simulink model "One_Phase_Controlled_Thyristor_Rectifier"  (R2015a)
settings: Solver=ode45  StartTime=0.0  StopTime=1  RelTol=1e-3
libraries: powerlib x29, powerlib_meascontrol x6
settings Model: Creator=Koustubh  LastModifiedBy=Koustubh

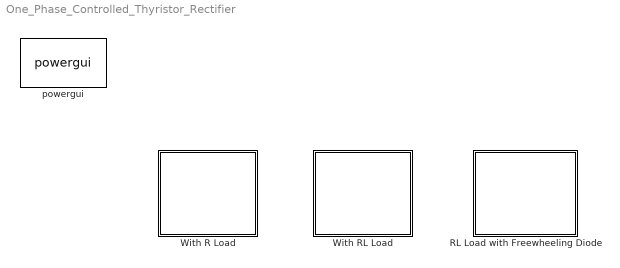
== system One_Phase_Controlled_Thyristor_Rectifier ==
  RL Load with Freewheeling Diode : Subsystem
  With R Load : Subsystem
  With RL Load : Subsystem
  powergui : powerlib/powergui  Priority=1  SimulationMode=Discrete  SolverType=Tustin/Backward Euler (TBE)  SampleTime=50e-6  frequency=60  SPID=off  DisableSnubberDevices=off  DisableRonSwitches=off  DisableVfSwitches=off  SwTol=0  DisplayEquations=off  Interpol=off  methode=off  Ts=100  FunctionMessages=off  echomessages=off  HookPort=off  EnableUseOfTLC=off  x0status=blocks  frequencyindice=50  Pbase=100e6  ErrMax=1e-4  Iterations=50  UnitsV=kV  UnitsW=MW  buscounter=0  RestoreLinks=warning  ResistiveCurrentMeasurement=off  Frange=[0:2:500]  Ylog=off  Xlog=on  ShowGrid=off  save=off  variable=ZData  structure=0  ZoomFFT=off  StartTime=0.0  cycles=1  DisplayStyle=1  fundamental=60  FreqAxis=off  MaxFrequency=1000  frequencyindicesteady=1  RmsSteady=1  display=off

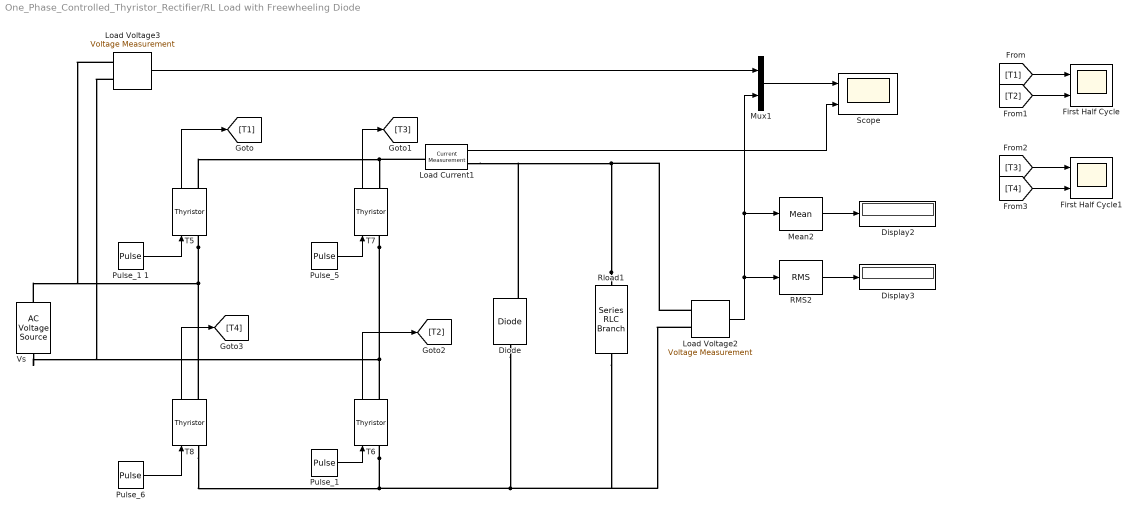
== system One_Phase_Controlled_Thyristor_Rectifier/RL Load with Freewheeling Diode ==
  Diode : powerlib/Power Electronics/Diode  Ron=0.001  Lon=0  Vf=0.8  IC=0  UseSnubber=off  Rs=500  Cs=250e-9  Measurements=on
  Display2 : Display
  Display3 : Display
  First Half Cycle : Scope  NumInputPorts=2
      settings: YMin=-5~-5  YMax=5~5  SaveName=ScopeData7
  First Half Cycle1 : Scope  NumInputPorts=2
      settings: YMin=-5~-5  YMax=5~5  SaveName=ScopeData8
  Load Current1 : powerlib/Measurements/Current Measurement  PhasorSimulation=off  OutputType=Complex  PSBequivalent=0
  Load Voltage2 : powerlib/Measurements/Voltage Measurement  PhasorSimulation=off  OutputType=Complex  PSBequivalent=0
  Load Voltage3 : powerlib/Measurements/Voltage Measurement  PhasorSimulation=off  OutputType=Complex  PSBequivalent=0
  Mean2 : powerlib_meascontrol/Measurements/Mean  Freq=50  Vinit=0  Ts=0
  Mux1 : Mux  Inputs=2
  Pulse_1 : DiscretePulseGenerator  PulseType=Time based  Period=0.02  PulseWidth=5  PhaseDelay=0.0025
  Pulse_1 1 : DiscretePulseGenerator  PulseType=Time based  Period=0.02  PulseWidth=5  PhaseDelay=0.0025
  Pulse_5 : DiscretePulseGenerator  PulseType=Time based  Period=0.02  PulseWidth=5  PhaseDelay=0.0125
  Pulse_6 : DiscretePulseGenerator  PulseType=Time based  Period=0.02  PulseWidth=5  PhaseDelay=0.0125
  RMS2 : powerlib_meascontrol/Measurements/RMS  TrueRMS=on  Freq=50  RMSInit=0  Ts=0
  Rload1 : powerlib/Elements/Series RLC Branch  LConnTagsString=__new0  RConnTagsString=__new0  BranchType=RL  Resistance=1  Inductance=1e-3  SetiL0=off  InitialCurrent=0  Capacitance=1e-6  Setx0=off  InitialVoltage=0  Measurements=None
  Scope : Scope  NumInputPorts=2
      settings: YMin=-5~-5  YMax=5~5  SaveName=ScopeData2
  T{5..8} (4 alike) : powerlib/Power Electronics/Thyristor  Ron=0.001  Lon=0  Vf=0.8  IC=0  Rs=500  Cs=250e-9  Measurements=on
  Vs : powerlib/Electrical Sources/AC Voltage Source  Amplitude=230*1.414  Phase=0  Frequency=50  SampleTime=0  Measurements=None
  wires:
  T7/1 -> [T3]
  T6/1 -> [T2]
  T5/1 -> [T1]
  T8/1 -> [T4]
  Pulse_1 1/1 -> T5/1
  Pulse_5/1 -> T7/1
  Pulse_1/1 -> T6/1
  Pulse_6/1 -> T8/1
  Load Voltage3/1 -> Mux1/1
  RMS2/1 -> Display3/1
  Load Voltage2/1 -> RMS2/1, Mean2/1, Mux1/2
  Mean2/1 -> Display2/1
  Load Current1/1 -> Scope/2
  Mux1/1 -> Scope/1
  [T1] -> First Half Cycle/1
  [T2] -> First Half Cycle/2
  [T3] -> First Half Cycle1/1
  [T4] -> First Half Cycle1/2
  connections:
  Rload1/LConn1 -- Diode/RConn1 -- Load Current1/RConn1 -- Load Voltage2/LConn1
  Load Current1/LConn1 -- T5/RConn1 -- T7/RConn1
  T6/LConn1 -- Diode/LConn1 -- Rload1/RConn1 -- Load Voltage2/LConn2 -- T8/LConn1
  T7/LConn1 -- T6/RConn1 -- Vs/LConn1 -- Load Voltage3/LConn2
  T5/LConn1 -- T8/RConn1 -- Vs/RConn1 -- Load Voltage3/LConn1

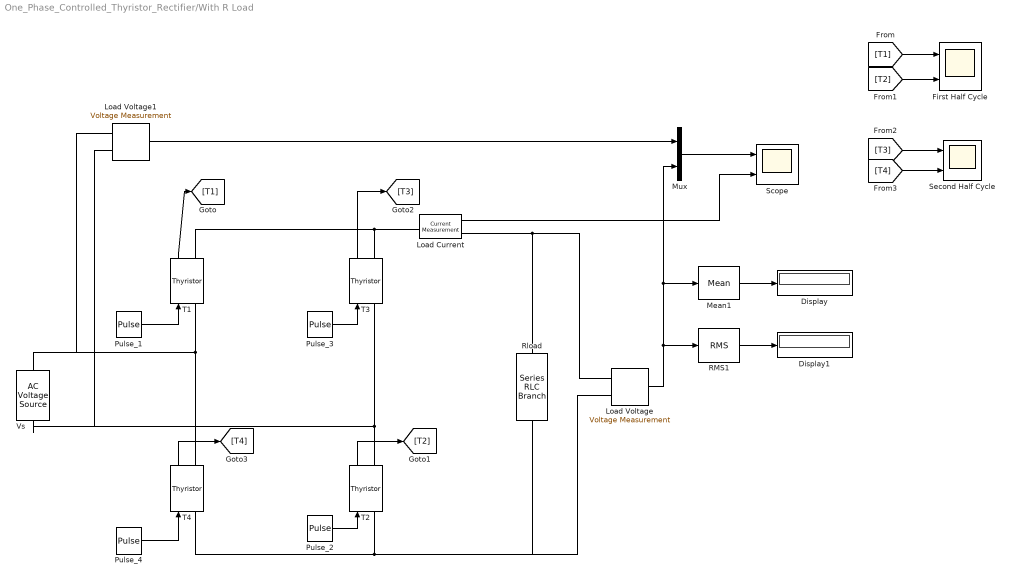
== system One_Phase_Controlled_Thyristor_Rectifier/With R Load ==
  Display : Display
  Display1 : Display
  First Half Cycle : Scope  NumInputPorts=2
      settings: YMin=-5~-5  YMax=5~5  SaveName=ScopeData3
  Load Current : powerlib/Measurements/Current Measurement  PhasorSimulation=off  OutputType=Complex  PSBequivalent=0
  Load Voltage : powerlib/Measurements/Voltage Measurement  PhasorSimulation=off  OutputType=Complex  PSBequivalent=0
  Load Voltage1 : powerlib/Measurements/Voltage Measurement  PhasorSimulation=off  OutputType=Complex  PSBequivalent=0
  Mean1 : powerlib_meascontrol/Measurements/Mean  Freq=50  Vinit=0  Ts=0
  Mux : Mux  Inputs=2
  "Pulse_1 " : DiscretePulseGenerator  PulseType=Time based  Period=0.02  PulseWidth=5  PhaseDelay=0.0025
  Pulse_2 : DiscretePulseGenerator  PulseType=Time based  Period=0.02  PulseWidth=5  PhaseDelay=0.0025
  Pulse_3 : DiscretePulseGenerator  PulseType=Time based  Period=0.02  PulseWidth=5  PhaseDelay=0.0125
  Pulse_4 : DiscretePulseGenerator  PulseType=Time based  Period=0.02  PulseWidth=5  PhaseDelay=0.0125
  RMS1 : powerlib_meascontrol/Measurements/RMS  TrueRMS=on  Freq=50  RMSInit=0  Ts=0
  Rload : powerlib/Elements/Series RLC Branch  LConnTagsString=__new0  RConnTagsString=__new0  BranchType=R  Resistance=10  Inductance=1e-3  SetiL0=off  InitialCurrent=0  Capacitance=1e-6  Setx0=off  InitialVoltage=0  Measurements=None
  Scope : Scope  NumInputPorts=2
      settings: YMin=-5~-5  YMax=5~5
  Second Half Cycle : Scope  NumInputPorts=2
      settings: YMin=-5~-5  YMax=5~5  SaveName=ScopeData4
  T{1..4} (4 alike) : powerlib/Power Electronics/Thyristor  Ron=0.001  Lon=0  Vf=0.8  IC=0  Rs=500  Cs=250e-9  Measurements=on
  Vs : powerlib/Electrical Sources/AC Voltage Source  Amplitude=230*1.414  Phase=0  Frequency=50  SampleTime=0  Measurements=None
  wires:
  Mean1/1 -> Display/1
  Mux/1 -> Scope/1
  "Pulse_1 "/1 -> T1/1
  Pulse_2/1 -> T2/1
  RMS1/1 -> Display1/1
  Pulse_4/1 -> T4/1
  Load Voltage/1 -> RMS1/1, Mean1/1, Mux/2
  Load Current/1 -> Scope/2
  Load Voltage1/1 -> Mux/1
  Pulse_3/1 -> T3/1
  T3/1 -> [T3]
  T4/1 -> [T4]
  T1/1 -> [T1]
  T2/1 -> [T2]
  [T1] -> First Half Cycle/1
  [T2] -> First Half Cycle/2
  [T3] -> Second Half Cycle/1
  [T4] -> Second Half Cycle/2
  connections:
  T2/RConn1 -- Vs/LConn1 -- Load Voltage1/LConn2 -- T3/LConn1
  T1/RConn1 -- T3/RConn1 -- Load Current/LConn1
  Load Current/RConn1 -- Load Voltage/LConn1 -- Rload/LConn1
  T4/RConn1 -- Vs/RConn1 -- Load Voltage1/LConn1 -- T1/LConn1
  T4/LConn1 -- Rload/RConn1 -- Load Voltage/LConn2 -- T2/LConn1

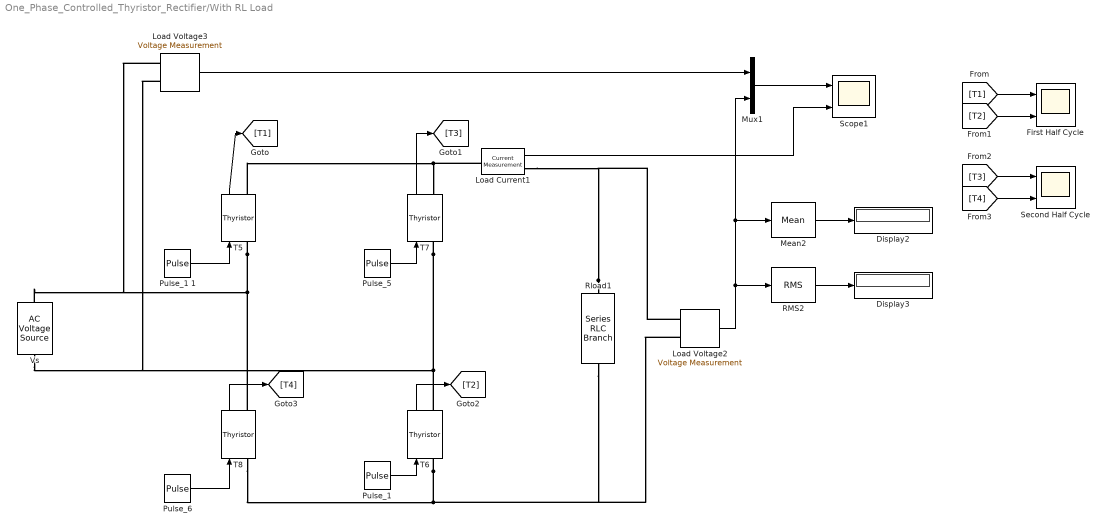
== system One_Phase_Controlled_Thyristor_Rectifier/With RL Load ==
  Display2 : Display
  Display3 : Display
  First Half Cycle : Scope  NumInputPorts=2
      settings: YMin=-5~-5  YMax=5~5  SaveName=ScopeData5
  Load Current1 : powerlib/Measurements/Current Measurement  PhasorSimulation=off  OutputType=Complex  PSBequivalent=0
  Load Voltage2 : powerlib/Measurements/Voltage Measurement  PhasorSimulation=off  OutputType=Complex  PSBequivalent=0
  Load Voltage3 : powerlib/Measurements/Voltage Measurement  PhasorSimulation=off  OutputType=Complex  PSBequivalent=0
  Mean2 : powerlib_meascontrol/Measurements/Mean  Freq=50  Vinit=0  Ts=0
  Mux1 : Mux  Inputs=2
  Pulse_1 : DiscretePulseGenerator  PulseType=Time based  Period=0.02  PulseWidth=5  PhaseDelay=0.0025
  Pulse_1 1 : DiscretePulseGenerator  PulseType=Time based  Period=0.02  PulseWidth=5  PhaseDelay=0.0025
  Pulse_5 : DiscretePulseGenerator  PulseType=Time based  Period=0.02  PulseWidth=5  PhaseDelay=0.0125
  Pulse_6 : DiscretePulseGenerator  PulseType=Time based  Period=0.02  PulseWidth=5  PhaseDelay=0.0125
  RMS2 : powerlib_meascontrol/Measurements/RMS  TrueRMS=on  Freq=50  RMSInit=0  Ts=0
  Rload1 : powerlib/Elements/Series RLC Branch  LConnTagsString=__new0  RConnTagsString=__new0  BranchType=RL  Resistance=1  Inductance=1e-3  SetiL0=off  InitialCurrent=0  Capacitance=1e-6  Setx0=off  InitialVoltage=0  Measurements=None
  Scope1 : Scope  NumInputPorts=2
      settings: YMin=-5~-5  YMax=5~5
  Second Half Cycle : Scope  NumInputPorts=2
      settings: YMin=-5~-5  YMax=5~5  SaveName=ScopeData6
  T{5..8} (4 alike) : powerlib/Power Electronics/Thyristor  Ron=0.001  Lon=0  Vf=0.8  IC=0  Rs=500  Cs=250e-9  Measurements=on
  Vs : powerlib/Electrical Sources/AC Voltage Source  Amplitude=230*1.414  Phase=0  Frequency=50  SampleTime=0  Measurements=None
  wires:
  Pulse_5/1 -> T7/1
  Pulse_1/1 -> T6/1
  Pulse_1 1/1 -> T5/1
  Pulse_6/1 -> T8/1
  Load Voltage3/1 -> Mux1/1
  RMS2/1 -> Display3/1
  Mean2/1 -> Display2/1
  Mux1/1 -> Scope1/1
  Load Voltage2/1 -> RMS2/1, Mean2/1, Mux1/2
  Load Current1/1 -> Scope1/2
  T8/1 -> [T4]
  T7/1 -> [T3]
  T6/1 -> [T2]
  T5/1 -> [T1]
  [T1] -> First Half Cycle/1
  [T2] -> First Half Cycle/2
  [T3] -> Second Half Cycle/1
  [T4] -> Second Half Cycle/2
  connections:
  Rload1/LConn1 -- Load Current1/RConn1 -- Load Voltage2/LConn1
  T6/LConn1 -- T8/LConn1 -- Rload1/RConn1 -- Load Voltage2/LConn2
  Load Current1/LConn1 -- T5/RConn1 -- T7/RConn1
  T7/LConn1 -- T6/RConn1 -- Vs/LConn1 -- Load Voltage3/LConn2
  T5/LConn1 -- T8/RConn1 -- Vs/RConn1 -- Load Voltage3/LConn1
